simulink model "final_test1"  (Simulink 7.7)
settings: Solver=ode45  StartTime=0.0  StopTime=10.0  RelTol=1e-3
undefined symbols (not defined in the file): des_attributefunction_support, des_figposition
libraries: simeventsattributes2 x107, simeventsserver1 x73, simeventstranslate1 x43, simeventsrouting1 x28, commrandsrc2 x18, simeventsgenerators1 x12, simeventssink1 x9, simeventsqueue1 x6, simulink_extras x1, simeventssignalmanage1 x1
(part 1 of 5)
settings Model: Creator=german  LastModifiedBy=german
settings SimEventsCC: propDiagAttribOutput=1  propDiagFcnCallOutput=1  propDiagStatOutput=0  propDiagChangeAttrib=0

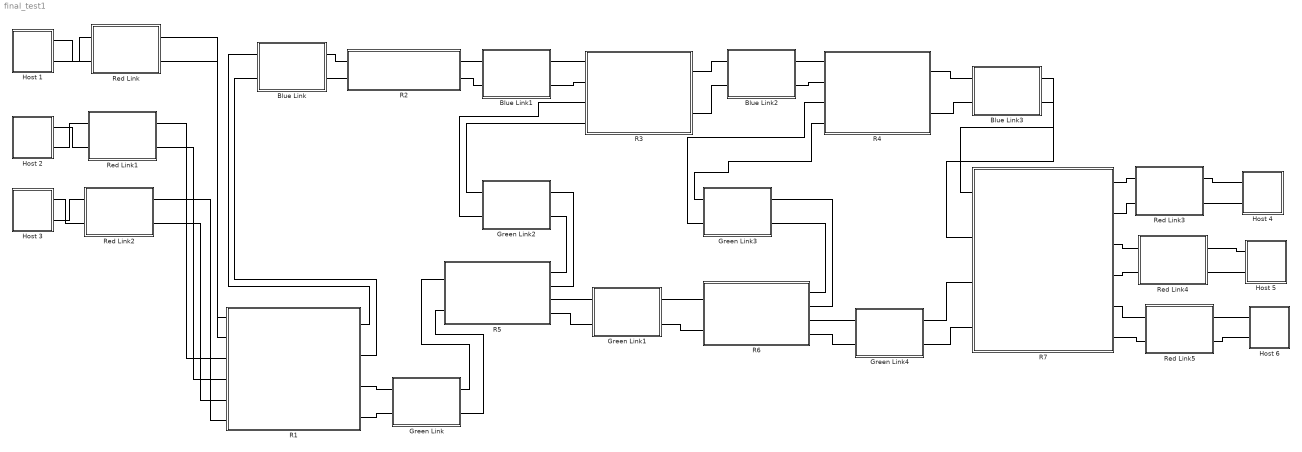
== system final_test1 ==
  Blue Link : Subsystem
  Blue Link1 : Subsystem
  Blue Link2 : Subsystem
  Blue Link3 : Subsystem
  Green Link : Subsystem
  Green Link1 : Subsystem
  Green Link2 : Subsystem
  Green Link3 : Subsystem
  Green Link4 : Subsystem
  Host 1 : Subsystem
  Host 2 : Subsystem
  Host 3 : Subsystem
  Host 4 : Subsystem
  Host 5 : Subsystem
  Host 6 : Subsystem
  R1 : Subsystem
  R2 : Subsystem
  R3 : Subsystem
  R4 : Subsystem
  R5 : Subsystem
  R6 : Subsystem
  R7 : Subsystem
  Red Link : Subsystem
  Red Link1 : Subsystem
  Red Link2 : Subsystem
  Red Link3 : Subsystem
  Red Link4 : Subsystem
  Red Link5 : Subsystem
  connections:
  Red Link/LConn2 -- Host 1/RConn1
  Host 1/RConn2 -- Red Link/LConn1
  Red Link/RConn1 -- R1/LConn1
  R1/LConn2 -- Red Link/RConn2
  Host 2/RConn2 -- Red Link1/LConn1
  Host 2/RConn1 -- Red Link1/LConn2
  Red Link1/RConn1 -- R1/LConn3
  R1/LConn4 -- Red Link1/RConn2
  Host 3/RConn2 -- Red Link2/LConn1
  Red Link2/LConn2 -- Host 3/RConn1
  Red Link2/RConn1 -- R1/LConn6
  Red Link2/RConn2 -- R1/LConn5
  Red Link3/RConn1 -- Host 4/LConn1
  Host 4/LConn2 -- Red Link3/RConn2
  Red Link4/RConn1 -- Host 5/LConn1
  Host 5/LConn2 -- Red Link4/RConn2
  Red Link5/RConn1 -- Host 6/LConn1
  Host 6/LConn2 -- Red Link5/RConn2
  Red Link5/LConn2 -- R7/RConn6
  Red Link5/LConn1 -- R7/RConn5
  Red Link4/LConn2 -- R7/RConn4
  Red Link4/LConn1 -- R7/RConn3
  Red Link3/LConn2 -- R7/RConn2
  Red Link3/LConn1 -- R7/RConn1
  R1/RConn1 -- Blue Link/LConn1
  Blue Link/LConn2 -- R1/RConn2
  Blue Link/RConn1 -- R2/LConn1
  R2/LConn2 -- Blue Link/RConn2
  Blue Link1/RConn1 -- R3/LConn1
  R2/RConn1 -- Blue Link1/LConn1
  R2/RConn2 -- Blue Link1/LConn2
  Blue Link1/RConn2 -- R3/LConn2
  Blue Link2/LConn2 -- R3/RConn2
  Blue Link2/LConn1 -- R3/RConn1
  Blue Link2/RConn1 -- R4/LConn1
  Blue Link2/RConn2 -- R4/LConn2
  R4/RConn1 -- Blue Link3/LConn1
  Blue Link3/LConn2 -- R4/RConn2
  R7/LConn1 -- Blue Link3/RConn1
  Blue Link3/RConn2 -- R7/LConn2
  Green Link/RConn1 -- R5/LConn1
  R1/RConn3 -- Green Link/LConn1
  Green Link/RConn2 -- R5/LConn2
  Green Link/LConn2 -- R1/RConn4
  R5/RConn1 -- Green Link2/RConn2
  R5/RConn2 -- Green Link2/RConn1
  Green Link2/LConn1 -- R3/LConn4
  R3/LConn3 -- Green Link2/LConn2
  R5/RConn3 -- Green Link1/LConn1
  R5/RConn4 -- Green Link1/LConn2
  Green Link1/RConn1 -- R6/LConn1
  Green Link1/RConn2 -- R6/LConn2
  R6/RConn1 -- Green Link3/RConn2
  R6/RConn2 -- Green Link3/RConn1
  Green Link3/LConn1 -- R4/LConn4
  Green Link3/LConn2 -- R4/LConn3
  R6/RConn3 -- Green Link4/LConn1
  R6/RConn4 -- Green Link4/LConn2
  Green Link4/RConn1 -- R7/LConn3
  R7/LConn4 -- Green Link4/RConn2

== system final_test1/Blue Link ==
  Attribute Function : Subsystem  LoadFcn=des_attributefunction_support(gcb,'LoadFcn');  StartFcn=des_attributefunction_support(gcb,'StartFcn');  mask(Attribute Function){OutputNamePrefix=out_}
      mask prompts: OutputNamePrefix "Prefix name"
      settings: CopyFcn=des_attributefunction_support(gcb,'CopyFcn');  OpenFcn=des_attributefunction_support(gcb,'OpenFcn');  ErrorFcn=des_error_redirect
      mask Help: helpview(simeventsbhelp('attributefunction'))
      mask Display: image(des_iconLoad('attribFunction.jpg'),'center');
  Attribute Function1 : Subsystem  LoadFcn=des_attributefunction_support(gcb,'LoadFcn');  StartFcn=des_attributefunction_support(gcb,'StartFcn');  mask(Attribute Function){OutputNamePrefix=out_}
      mask prompts: OutputNamePrefix "Prefix name"
      settings: CopyFcn=des_attributefunction_support(gcb,'CopyFcn');  OpenFcn=des_attributefunction_support(gcb,'OpenFcn');  ErrorFcn=des_error_redirect
      mask Help: helpview(simeventsbhelp('attributefunction'))
      mask Display: image(des_iconLoad('attribFunction.jpg'),'center');
  Infinite Server : simeventsserver1/Infinite Server  SystemSampleTime=-1  ServiceTimeFrom=Dialog  ServiceTime=0.007  AttributeName=ServiceTime  PriorityServiceCompletion=500  EnableTOPort=off  StatNumberDeparted=Off  StatNumberInBlock=Off  StatPendingEntity=Off  StatNumberPending=Off  StatAverageWait=Off  StatNumberTimedout=Off
  Infinite Server1 : simeventsserver1/Infinite Server  SystemSampleTime=-1  ServiceTimeFrom=Dialog  ServiceTime=0.007  AttributeName=ServiceTime  PriorityServiceCompletion=500  EnableTOPort=off  StatNumberDeparted=Off  StatNumberInBlock=Off  StatPendingEntity=Off  StatNumberPending=Off  StatAverageWait=Off  StatNumberTimedout=Off
  Single Server : simeventsserver1/Single Server  SystemSampleTime=-1  ServiceTimeFrom=Attribute  ServiceTime=1  AttributeName=ServiceTime  PriorityServiceCompletion=500  PermitPreemption=off  SortingAttributeName=PriorityAttributeName  SortingDirection=Ascending  WriteToAttribute=off  ResidualAttributeName=ResidualServiceTime  CreateAttribute=on  EnableTOPort=off  StatNumberDeparted=Off  StatNumberInBlock=Off  StatNumberPreempted=Off  StatPendingEntity=Off  StatAverageWait=Off  StatUtilization=Off  StatNumberTimedout=Off
  Single Server1 : simeventsserver1/Single Server  SystemSampleTime=-1  ServiceTimeFrom=Attribute  ServiceTime=1  AttributeName=ServiceTime  PriorityServiceCompletion=500  PermitPreemption=off  SortingAttributeName=PriorityAttributeName  SortingDirection=Ascending  WriteToAttribute=off  ResidualAttributeName=ResidualServiceTime  CreateAttribute=on  EnableTOPort=off  StatNumberDeparted=Off  StatNumberInBlock=Off  StatNumberPreempted=Off  StatPendingEntity=Off  StatAverageWait=Off  StatUtilization=Off  StatNumberTimedout=Off
  Input1 : PMIOPort  Port=1  Side=Left
  Output1 : PMIOPort  Port=2  Side=Right
  Input2 : PMIOPort  Port=3  Side=Right
  Output2 : PMIOPort  Port=4  Side=Left
  connections:
  Attribute Function1/RConn1 -- Single Server1/LConn1
  Input2/RConn1 -- Attribute Function1/LConn1
  Single Server1/RConn1 -- Infinite Server/LConn1
  Single Server/RConn1 -- Infinite Server1/LConn1
  Attribute Function/RConn1 -- Single Server/LConn1
  Output2/RConn1 -- Infinite Server/RConn1
  Output1/RConn1 -- Infinite Server1/RConn1
  Input1/RConn1 -- Attribute Function/LConn1

== system final_test1/Blue Link1 ==
  Attribute Function : Subsystem  LoadFcn=des_attributefunction_support(gcb,'LoadFcn');  StartFcn=des_attributefunction_support(gcb,'StartFcn');  mask(Attribute Function){OutputNamePrefix=out_}
      mask prompts: OutputNamePrefix "Prefix name"
      settings: CopyFcn=des_attributefunction_support(gcb,'CopyFcn');  OpenFcn=des_attributefunction_support(gcb,'OpenFcn');  ErrorFcn=des_error_redirect
      mask Help: helpview(simeventsbhelp('attributefunction'))
      mask Display: image(des_iconLoad('attribFunction.jpg'),'center');
  Attribute Function1 : Subsystem  LoadFcn=des_attributefunction_support(gcb,'LoadFcn');  StartFcn=des_attributefunction_support(gcb,'StartFcn');  mask(Attribute Function){OutputNamePrefix=out_}
      mask prompts: OutputNamePrefix "Prefix name"
      settings: CopyFcn=des_attributefunction_support(gcb,'CopyFcn');  OpenFcn=des_attributefunction_support(gcb,'OpenFcn');  ErrorFcn=des_error_redirect
      mask Help: helpview(simeventsbhelp('attributefunction'))
      mask Display: image(des_iconLoad('attribFunction.jpg'),'center');
  Infinite Server : simeventsserver1/Infinite Server  SystemSampleTime=-1  ServiceTimeFrom=Dialog  ServiceTime=0.007  AttributeName=ServiceTime  PriorityServiceCompletion=500  EnableTOPort=off  StatNumberDeparted=Off  StatNumberInBlock=Off  StatPendingEntity=Off  StatNumberPending=Off  StatAverageWait=Off  StatNumberTimedout=Off
  Infinite Server1 : simeventsserver1/Infinite Server  SystemSampleTime=-1  ServiceTimeFrom=Dialog  ServiceTime=0.007  AttributeName=ServiceTime  PriorityServiceCompletion=500  EnableTOPort=off  StatNumberDeparted=Off  StatNumberInBlock=Off  StatPendingEntity=Off  StatNumberPending=Off  StatAverageWait=Off  StatNumberTimedout=Off
  Single Server : simeventsserver1/Single Server  SystemSampleTime=-1  ServiceTimeFrom=Attribute  ServiceTime=1  AttributeName=ServiceTime  PriorityServiceCompletion=500  PermitPreemption=off  SortingAttributeName=PriorityAttributeName  SortingDirection=Ascending  WriteToAttribute=off  ResidualAttributeName=ResidualServiceTime  CreateAttribute=on  EnableTOPort=off  StatNumberDeparted=Off  StatNumberInBlock=Off  StatNumberPreempted=Off  StatPendingEntity=Off  StatAverageWait=Off  StatUtilization=Off  StatNumberTimedout=Off
  Single Server1 : simeventsserver1/Single Server  SystemSampleTime=-1  ServiceTimeFrom=Attribute  ServiceTime=1  AttributeName=ServiceTime  PriorityServiceCompletion=500  PermitPreemption=off  SortingAttributeName=PriorityAttributeName  SortingDirection=Ascending  WriteToAttribute=off  ResidualAttributeName=ResidualServiceTime  CreateAttribute=on  EnableTOPort=off  StatNumberDeparted=Off  StatNumberInBlock=Off  StatNumberPreempted=Off  StatPendingEntity=Off  StatAverageWait=Off  StatUtilization=Off  StatNumberTimedout=Off
  Input1 : PMIOPort  Port=1  Side=Left
  Output1 : PMIOPort  Port=2  Side=Right
  Input2 : PMIOPort  Port=3  Side=Right
  Output2 : PMIOPort  Port=4  Side=Left
  connections:
  Input1/RConn1 -- Attribute Function/LConn1
  Output1/RConn1 -- Infinite Server1/RConn1
  Output2/RConn1 -- Infinite Server/RConn1
  Attribute Function/RConn1 -- Single Server/LConn1
  Single Server/RConn1 -- Infinite Server1/LConn1
  Single Server1/RConn1 -- Infinite Server/LConn1
  Input2/RConn1 -- Attribute Function1/LConn1
  Attribute Function1/RConn1 -- Single Server1/LConn1

== system final_test1/Blue Link2 ==
  Attribute Function : Subsystem  LoadFcn=des_attributefunction_support(gcb,'LoadFcn');  StartFcn=des_attributefunction_support(gcb,'StartFcn');  mask(Attribute Function){OutputNamePrefix=out_}
      mask prompts: OutputNamePrefix "Prefix name"
      settings: CopyFcn=des_attributefunction_support(gcb,'CopyFcn');  OpenFcn=des_attributefunction_support(gcb,'OpenFcn');  ErrorFcn=des_error_redirect
      mask Help: helpview(simeventsbhelp('attributefunction'))
      mask Display: image(des_iconLoad('attribFunction.jpg'),'center');
  Attribute Function1 : Subsystem  LoadFcn=des_attributefunction_support(gcb,'LoadFcn');  StartFcn=des_attributefunction_support(gcb,'StartFcn');  mask(Attribute Function){OutputNamePrefix=out_}
      mask prompts: OutputNamePrefix "Prefix name"
      settings: CopyFcn=des_attributefunction_support(gcb,'CopyFcn');  OpenFcn=des_attributefunction_support(gcb,'OpenFcn');  ErrorFcn=des_error_redirect
      mask Help: helpview(simeventsbhelp('attributefunction'))
      mask Display: image(des_iconLoad('attribFunction.jpg'),'center');
  Infinite Server : simeventsserver1/Infinite Server  SystemSampleTime=-1  ServiceTimeFrom=Dialog  ServiceTime=0.007  AttributeName=ServiceTime  PriorityServiceCompletion=500  EnableTOPort=off  StatNumberDeparted=Off  StatNumberInBlock=Off  StatPendingEntity=Off  StatNumberPending=Off  StatAverageWait=Off  StatNumberTimedout=Off
  Infinite Server1 : simeventsserver1/Infinite Server  SystemSampleTime=-1  ServiceTimeFrom=Dialog  ServiceTime=0.007  AttributeName=ServiceTime  PriorityServiceCompletion=500  EnableTOPort=off  StatNumberDeparted=Off  StatNumberInBlock=Off  StatPendingEntity=Off  StatNumberPending=Off  StatAverageWait=Off  StatNumberTimedout=Off
  Single Server : simeventsserver1/Single Server  SystemSampleTime=-1  ServiceTimeFrom=Attribute  ServiceTime=1  AttributeName=ServiceTime  PriorityServiceCompletion=500  PermitPreemption=off  SortingAttributeName=PriorityAttributeName  SortingDirection=Ascending  WriteToAttribute=off  ResidualAttributeName=ResidualServiceTime  CreateAttribute=on  EnableTOPort=off  StatNumberDeparted=Off  StatNumberInBlock=Off  StatNumberPreempted=Off  StatPendingEntity=Off  StatAverageWait=Off  StatUtilization=Off  StatNumberTimedout=Off
  Single Server1 : simeventsserver1/Single Server  SystemSampleTime=-1  ServiceTimeFrom=Attribute  ServiceTime=1  AttributeName=ServiceTime  PriorityServiceCompletion=500  PermitPreemption=off  SortingAttributeName=PriorityAttributeName  SortingDirection=Ascending  WriteToAttribute=off  ResidualAttributeName=ResidualServiceTime  CreateAttribute=on  EnableTOPort=off  StatNumberDeparted=Off  StatNumberInBlock=Off  StatNumberPreempted=Off  StatPendingEntity=Off  StatAverageWait=Off  StatUtilization=Off  StatNumberTimedout=Off
  Input1 : PMIOPort  Port=1  Side=Left
  Output1 : PMIOPort  Port=2  Side=Right
  Input2 : PMIOPort  Port=3  Side=Right
  Output2 : PMIOPort  Port=4  Side=Left
  connections:
  Attribute Function1/RConn1 -- Single Server1/LConn1
  Input2/RConn1 -- Attribute Function1/LConn1
  Single Server1/RConn1 -- Infinite Server/LConn1
  Single Server/RConn1 -- Infinite Server1/LConn1
  Attribute Function/RConn1 -- Single Server/LConn1
  Output2/RConn1 -- Infinite Server/RConn1
  Output1/RConn1 -- Infinite Server1/RConn1
  Input1/RConn1 -- Attribute Function/LConn1

== system final_test1/Blue Link3 ==
  Attribute Function : Subsystem  LoadFcn=des_attributefunction_support(gcb,'LoadFcn');  StartFcn=des_attributefunction_support(gcb,'StartFcn');  mask(Attribute Function){OutputNamePrefix=out_}
      mask prompts: OutputNamePrefix "Prefix name"
      settings: CopyFcn=des_attributefunction_support(gcb,'CopyFcn');  OpenFcn=des_attributefunction_support(gcb,'OpenFcn');  ErrorFcn=des_error_redirect
      mask Help: helpview(simeventsbhelp('attributefunction'))
      mask Display: image(des_iconLoad('attribFunction.jpg'),'center');
  Attribute Function1 : Subsystem  LoadFcn=des_attributefunction_support(gcb,'LoadFcn');  StartFcn=des_attributefunction_support(gcb,'StartFcn');  mask(Attribute Function){OutputNamePrefix=out_}
      mask prompts: OutputNamePrefix "Prefix name"
      settings: CopyFcn=des_attributefunction_support(gcb,'CopyFcn');  OpenFcn=des_attributefunction_support(gcb,'OpenFcn');  ErrorFcn=des_error_redirect
      mask Help: helpview(simeventsbhelp('attributefunction'))
      mask Display: image(des_iconLoad('attribFunction.jpg'),'center');
  Infinite Server : simeventsserver1/Infinite Server  SystemSampleTime=-1  ServiceTimeFrom=Dialog  ServiceTime=0.007  AttributeName=ServiceTime  PriorityServiceCompletion=500  EnableTOPort=off  StatNumberDeparted=Off  StatNumberInBlock=Off  StatPendingEntity=Off  StatNumberPending=Off  StatAverageWait=Off  StatNumberTimedout=Off
  Infinite Server1 : simeventsserver1/Infinite Server  SystemSampleTime=-1  ServiceTimeFrom=Dialog  ServiceTime=0.007  AttributeName=ServiceTime  PriorityServiceCompletion=500  EnableTOPort=off  StatNumberDeparted=Off  StatNumberInBlock=Off  StatPendingEntity=Off  StatNumberPending=Off  StatAverageWait=Off  StatNumberTimedout=Off
  Single Server : simeventsserver1/Single Server  SystemSampleTime=-1  ServiceTimeFrom=Attribute  ServiceTime=1  AttributeName=ServiceTime  PriorityServiceCompletion=500  PermitPreemption=off  SortingAttributeName=PriorityAttributeName  SortingDirection=Ascending  WriteToAttribute=off  ResidualAttributeName=ResidualServiceTime  CreateAttribute=on  EnableTOPort=off  StatNumberDeparted=Off  StatNumberInBlock=Off  StatNumberPreempted=Off  StatPendingEntity=Off  StatAverageWait=Off  StatUtilization=Off  StatNumberTimedout=Off
  Single Server1 : simeventsserver1/Single Server  SystemSampleTime=-1  ServiceTimeFrom=Attribute  ServiceTime=1  AttributeName=ServiceTime  PriorityServiceCompletion=500  PermitPreemption=off  SortingAttributeName=PriorityAttributeName  SortingDirection=Ascending  WriteToAttribute=off  ResidualAttributeName=ResidualServiceTime  CreateAttribute=on  EnableTOPort=off  StatNumberDeparted=Off  StatNumberInBlock=Off  StatNumberPreempted=Off  StatPendingEntity=Off  StatAverageWait=Off  StatUtilization=Off  StatNumberTimedout=Off
  Input1 : PMIOPort  Port=1  Side=Left
  Output1 : PMIOPort  Port=2  Side=Right
  Input2 : PMIOPort  Port=3  Side=Right
  Output2 : PMIOPort  Port=4  Side=Left
  connections:
  Input1/RConn1 -- Attribute Function/LConn1
  Output1/RConn1 -- Infinite Server1/RConn1
  Output2/RConn1 -- Infinite Server/RConn1
  Attribute Function/RConn1 -- Single Server/LConn1
  Single Server/RConn1 -- Infinite Server1/LConn1
  Single Server1/RConn1 -- Infinite Server/LConn1
  Input2/RConn1 -- Attribute Function1/LConn1
  Attribute Function1/RConn1 -- Single Server1/LConn1

== system final_test1/Green Link ==
  Attribute Function : Subsystem  LoadFcn=des_attributefunction_support(gcb,'LoadFcn');  StartFcn=des_attributefunction_support(gcb,'StartFcn');  mask(Attribute Function){OutputNamePrefix=out_}
      mask prompts: OutputNamePrefix "Prefix name"
      settings: CopyFcn=des_attributefunction_support(gcb,'CopyFcn');  OpenFcn=des_attributefunction_support(gcb,'OpenFcn');  ErrorFcn=des_error_redirect
      mask Help: helpview(simeventsbhelp('attributefunction'))
      mask Display: image(des_iconLoad('attribFunction.jpg'),'center');
  Attribute Function1 : Subsystem  LoadFcn=des_attributefunction_support(gcb,'LoadFcn');  StartFcn=des_attributefunction_support(gcb,'StartFcn');  mask(Attribute Function){OutputNamePrefix=out_}
      mask prompts: OutputNamePrefix "Prefix name"
      settings: CopyFcn=des_attributefunction_support(gcb,'CopyFcn');  OpenFcn=des_attributefunction_support(gcb,'OpenFcn');  ErrorFcn=des_error_redirect
      mask Help: helpview(simeventsbhelp('attributefunction'))
      mask Display: image(des_iconLoad('attribFunction.jpg'),'center');
  Infinite Server : simeventsserver1/Infinite Server  SystemSampleTime=-1  ServiceTimeFrom=Dialog  ServiceTime=0.003  AttributeName=ServiceTime  PriorityServiceCompletion=500  EnableTOPort=off  StatNumberDeparted=Off  StatNumberInBlock=Off  StatPendingEntity=Off  StatNumberPending=Off  StatAverageWait=Off  StatNumberTimedout=Off
  Infinite Server1 : simeventsserver1/Infinite Server  SystemSampleTime=-1  ServiceTimeFrom=Dialog  ServiceTime=0.003  AttributeName=ServiceTime  PriorityServiceCompletion=500  EnableTOPort=off  StatNumberDeparted=Off  StatNumberInBlock=Off  StatPendingEntity=Off  StatNumberPending=Off  StatAverageWait=Off  StatNumberTimedout=Off
  Single Server : simeventsserver1/Single Server  SystemSampleTime=-1  ServiceTimeFrom=Attribute  ServiceTime=1  AttributeName=ServiceTime  PriorityServiceCompletion=500  PermitPreemption=off  SortingAttributeName=PriorityAttributeName  SortingDirection=Ascending  WriteToAttribute=off  ResidualAttributeName=ResidualServiceTime  CreateAttribute=on  EnableTOPort=off  StatNumberDeparted=Off  StatNumberInBlock=Off  StatNumberPreempted=Off  StatPendingEntity=Off  StatAverageWait=Off  StatUtilization=Off  StatNumberTimedout=Off
  Single Server1 : simeventsserver1/Single Server  SystemSampleTime=-1  ServiceTimeFrom=Attribute  ServiceTime=1  AttributeName=ServiceTime  PriorityServiceCompletion=500  PermitPreemption=off  SortingAttributeName=PriorityAttributeName  SortingDirection=Ascending  WriteToAttribute=off  ResidualAttributeName=ResidualServiceTime  CreateAttribute=on  EnableTOPort=off  StatNumberDeparted=Off  StatNumberInBlock=Off  StatNumberPreempted=Off  StatPendingEntity=Off  StatAverageWait=Off  StatUtilization=Off  StatNumberTimedout=Off
  Input1 : PMIOPort  Port=1  Side=Left
  Output1 : PMIOPort  Port=2  Side=Right
  Input2 : PMIOPort  Port=3  Side=Right
  Output2 : PMIOPort  Port=4  Side=Left
  connections:
  Attribute Function1/RConn1 -- Single Server1/LConn1
  Input2/RConn1 -- Attribute Function1/LConn1
  Single Server1/RConn1 -- Infinite Server/LConn1
  Single Server/RConn1 -- Infinite Server1/LConn1
  Attribute Function/RConn1 -- Single Server/LConn1
  Output2/RConn1 -- Infinite Server/RConn1
  Output1/RConn1 -- Infinite Server1/RConn1
  Input1/RConn1 -- Attribute Function/LConn1

== system final_test1/Green Link1 ==
  Attribute Function : Subsystem  LoadFcn=des_attributefunction_support(gcb,'LoadFcn');  StartFcn=des_attributefunction_support(gcb,'StartFcn');  mask(Attribute Function){OutputNamePrefix=out_}
      mask prompts: OutputNamePrefix "Prefix name"
      settings: CopyFcn=des_attributefunction_support(gcb,'CopyFcn');  OpenFcn=des_attributefunction_support(gcb,'OpenFcn');  ErrorFcn=des_error_redirect
      mask Help: helpview(simeventsbhelp('attributefunction'))
      mask Display: image(des_iconLoad('attribFunction.jpg'),'center');
  Attribute Function1 : Subsystem  LoadFcn=des_attributefunction_support(gcb,'LoadFcn');  StartFcn=des_attributefunction_support(gcb,'StartFcn');  mask(Attribute Function){OutputNamePrefix=out_}
      mask prompts: OutputNamePrefix "Prefix name"
      settings: CopyFcn=des_attributefunction_support(gcb,'CopyFcn');  OpenFcn=des_attributefunction_support(gcb,'OpenFcn');  ErrorFcn=des_error_redirect
      mask Help: helpview(simeventsbhelp('attributefunction'))
      mask Display: image(des_iconLoad('attribFunction.jpg'),'center');
  Infinite Server : simeventsserver1/Infinite Server  SystemSampleTime=-1  ServiceTimeFrom=Dialog  ServiceTime=0.003  AttributeName=ServiceTime  PriorityServiceCompletion=500  EnableTOPort=off  StatNumberDeparted=Off  StatNumberInBlock=Off  StatPendingEntity=Off  StatNumberPending=Off  StatAverageWait=Off  StatNumberTimedout=Off
  Infinite Server1 : simeventsserver1/Infinite Server  SystemSampleTime=-1  ServiceTimeFrom=Dialog  ServiceTime=0.003  AttributeName=ServiceTime  PriorityServiceCompletion=500  EnableTOPort=off  StatNumberDeparted=Off  StatNumberInBlock=Off  StatPendingEntity=Off  StatNumberPending=Off  StatAverageWait=Off  StatNumberTimedout=Off
  Single Server : simeventsserver1/Single Server  SystemSampleTime=-1  ServiceTimeFrom=Attribute  ServiceTime=1  AttributeName=ServiceTime  PriorityServiceCompletion=500  PermitPreemption=off  SortingAttributeName=PriorityAttributeName  SortingDirection=Ascending  WriteToAttribute=off  ResidualAttributeName=ResidualServiceTime  CreateAttribute=on  EnableTOPort=off  StatNumberDeparted=Off  StatNumberInBlock=Off  StatNumberPreempted=Off  StatPendingEntity=Off  StatAverageWait=Off  StatUtilization=Off  StatNumberTimedout=Off
  Single Server1 : simeventsserver1/Single Server  SystemSampleTime=-1  ServiceTimeFrom=Attribute  ServiceTime=1  AttributeName=ServiceTime  PriorityServiceCompletion=500  PermitPreemption=off  SortingAttributeName=PriorityAttributeName  SortingDirection=Ascending  WriteToAttribute=off  ResidualAttributeName=ResidualServiceTime  CreateAttribute=on  EnableTOPort=off  StatNumberDeparted=Off  StatNumberInBlock=Off  StatNumberPreempted=Off  StatPendingEntity=Off  StatAverageWait=Off  StatUtilization=Off  StatNumberTimedout=Off
  Input1 : PMIOPort  Port=1  Side=Left
  Output1 : PMIOPort  Port=2  Side=Right
  Input2 : PMIOPort  Port=3  Side=Right
  Output2 : PMIOPort  Port=4  Side=Left
  connections:
  Input1/RConn1 -- Attribute Function/LConn1
  Output1/RConn1 -- Infinite Server1/RConn1
  Output2/RConn1 -- Infinite Server/RConn1
  Attribute Function/RConn1 -- Single Server/LConn1
  Single Server/RConn1 -- Infinite Server1/LConn1
  Single Server1/RConn1 -- Infinite Server/LConn1
  Input2/RConn1 -- Attribute Function1/LConn1
  Attribute Function1/RConn1 -- Single Server1/LConn1

== system final_test1/Green Link2 ==
  Attribute Function : Subsystem  LoadFcn=des_attributefunction_support(gcb,'LoadFcn');  StartFcn=des_attributefunction_support(gcb,'StartFcn');  mask(Attribute Function){OutputNamePrefix=out_}
      mask prompts: OutputNamePrefix "Prefix name"
      settings: CopyFcn=des_attributefunction_support(gcb,'CopyFcn');  OpenFcn=des_attributefunction_support(gcb,'OpenFcn');  ErrorFcn=des_error_redirect
      mask Help: helpview(simeventsbhelp('attributefunction'))
      mask Display: image(des_iconLoad('attribFunction.jpg'),'center');
  Attribute Function1 : Subsystem  LoadFcn=des_attributefunction_support(gcb,'LoadFcn');  StartFcn=des_attributefunction_support(gcb,'StartFcn');  mask(Attribute Function){OutputNamePrefix=out_}
      mask prompts: OutputNamePrefix "Prefix name"
      settings: CopyFcn=des_attributefunction_support(gcb,'CopyFcn');  OpenFcn=des_attributefunction_support(gcb,'OpenFcn');  ErrorFcn=des_error_redirect
      mask Help: helpview(simeventsbhelp('attributefunction'))
      mask Display: image(des_iconLoad('attribFunction.jpg'),'center');
  Infinite Server : simeventsserver1/Infinite Server  SystemSampleTime=-1  ServiceTimeFrom=Dialog  ServiceTime=0.003  AttributeName=ServiceTime  PriorityServiceCompletion=500  EnableTOPort=off  StatNumberDeparted=Off  StatNumberInBlock=Off  StatPendingEntity=Off  StatNumberPending=Off  StatAverageWait=Off  StatNumberTimedout=Off
  Infinite Server1 : simeventsserver1/Infinite Server  SystemSampleTime=-1  ServiceTimeFrom=Dialog  ServiceTime=0.003  AttributeName=ServiceTime  PriorityServiceCompletion=500  EnableTOPort=off  StatNumberDeparted=Off  StatNumberInBlock=Off  StatPendingEntity=Off  StatNumberPending=Off  StatAverageWait=Off  StatNumberTimedout=Off
  Single Server : simeventsserver1/Single Server  SystemSampleTime=-1  ServiceTimeFrom=Attribute  ServiceTime=1  AttributeName=ServiceTime  PriorityServiceCompletion=500  PermitPreemption=off  SortingAttributeName=PriorityAttributeName  SortingDirection=Ascending  WriteToAttribute=off  ResidualAttributeName=ResidualServiceTime  CreateAttribute=on  EnableTOPort=off  StatNumberDeparted=Off  StatNumberInBlock=Off  StatNumberPreempted=Off  StatPendingEntity=Off  StatAverageWait=Off  StatUtilization=Off  StatNumberTimedout=Off
  Single Server1 : simeventsserver1/Single Server  SystemSampleTime=-1  ServiceTimeFrom=Attribute  ServiceTime=1  AttributeName=ServiceTime  PriorityServiceCompletion=500  PermitPreemption=off  SortingAttributeName=PriorityAttributeName  SortingDirection=Ascending  WriteToAttribute=off  ResidualAttributeName=ResidualServiceTime  CreateAttribute=on  EnableTOPort=off  StatNumberDeparted=Off  StatNumberInBlock=Off  StatNumberPreempted=Off  StatPendingEntity=Off  StatAverageWait=Off  StatUtilization=Off  StatNumberTimedout=Off
  Input1 : PMIOPort  Port=1  Side=Left
  Output1 : PMIOPort  Port=2  Side=Right
  Input2 : PMIOPort  Port=3  Side=Right
  Output2 : PMIOPort  Port=4  Side=Left
  connections:
  Attribute Function1/RConn1 -- Single Server1/LConn1
  Input2/RConn1 -- Attribute Function1/LConn1
  Single Server1/RConn1 -- Infinite Server/LConn1
  Single Server/RConn1 -- Infinite Server1/LConn1
  Attribute Function/RConn1 -- Single Server/LConn1
  Output2/RConn1 -- Infinite Server/RConn1
  Output1/RConn1 -- Infinite Server1/RConn1
  Input1/RConn1 -- Attribute Function/LConn1

== system final_test1/Green Link3 ==
  Attribute Function : Subsystem  LoadFcn=des_attributefunction_support(gcb,'LoadFcn');  StartFcn=des_attributefunction_support(gcb,'StartFcn');  mask(Attribute Function){OutputNamePrefix=out_}
      mask prompts: OutputNamePrefix "Prefix name"
      settings: CopyFcn=des_attributefunction_support(gcb,'CopyFcn');  OpenFcn=des_attributefunction_support(gcb,'OpenFcn');  ErrorFcn=des_error_redirect
      mask Help: helpview(simeventsbhelp('attributefunction'))
      mask Display: image(des_iconLoad('attribFunction.jpg'),'center');
  Attribute Function1 : Subsystem  LoadFcn=des_attributefunction_support(gcb,'LoadFcn');  StartFcn=des_attributefunction_support(gcb,'StartFcn');  mask(Attribute Function){OutputNamePrefix=out_}
      mask prompts: OutputNamePrefix "Prefix name"
      settings: CopyFcn=des_attributefunction_support(gcb,'CopyFcn');  OpenFcn=des_attributefunction_support(gcb,'OpenFcn');  ErrorFcn=des_error_redirect
      mask Help: helpview(simeventsbhelp('attributefunction'))
      mask Display: image(des_iconLoad('attribFunction.jpg'),'center');
  Infinite Server : simeventsserver1/Infinite Server  SystemSampleTime=-1  ServiceTimeFrom=Dialog  ServiceTime=0.003  AttributeName=ServiceTime  PriorityServiceCompletion=500  EnableTOPort=off  StatNumberDeparted=Off  StatNumberInBlock=Off  StatPendingEntity=Off  StatNumberPending=Off  StatAverageWait=Off  StatNumberTimedout=Off
  Infinite Server1 : simeventsserver1/Infinite Server  SystemSampleTime=-1  ServiceTimeFrom=Dialog  ServiceTime=0.003  AttributeName=ServiceTime  PriorityServiceCompletion=500  EnableTOPort=off  StatNumberDeparted=Off  StatNumberInBlock=Off  StatPendingEntity=Off  StatNumberPending=Off  StatAverageWait=Off  StatNumberTimedout=Off
  Single Server : simeventsserver1/Single Server  SystemSampleTime=-1  ServiceTimeFrom=Attribute  ServiceTime=1  AttributeName=ServiceTime  PriorityServiceCompletion=500  PermitPreemption=off  SortingAttributeName=PriorityAttributeName  SortingDirection=Ascending  WriteToAttribute=off  ResidualAttributeName=ResidualServiceTime  CreateAttribute=on  EnableTOPort=off  StatNumberDeparted=Off  StatNumberInBlock=Off  StatNumberPreempted=Off  StatPendingEntity=Off  StatAverageWait=Off  StatUtilization=Off  StatNumberTimedout=Off
  Single Server1 : simeventsserver1/Single Server  SystemSampleTime=-1  ServiceTimeFrom=Attribute  ServiceTime=1  AttributeName=ServiceTime  PriorityServiceCompletion=500  PermitPreemption=off  SortingAttributeName=PriorityAttributeName  SortingDirection=Ascending  WriteToAttribute=off  ResidualAttributeName=ResidualServiceTime  CreateAttribute=on  EnableTOPort=off  StatNumberDeparted=Off  StatNumberInBlock=Off  StatNumberPreempted=Off  StatPendingEntity=Off  StatAverageWait=Off  StatUtilization=Off  StatNumberTimedout=Off
  Input1 : PMIOPort  Port=1  Side=Left
  Output1 : PMIOPort  Port=2  Side=Right
  Input2 : PMIOPort  Port=3  Side=Right
  Output2 : PMIOPort  Port=4  Side=Left
  connections:
  Attribute Function1/RConn1 -- Single Server1/LConn1
  Input2/RConn1 -- Attribute Function1/LConn1
  Single Server1/RConn1 -- Infinite Server/LConn1
  Single Server/RConn1 -- Infinite Server1/LConn1
  Attribute Function/RConn1 -- Single Server/LConn1
  Output2/RConn1 -- Infinite Server/RConn1
  Output1/RConn1 -- Infinite Server1/RConn1
  Input1/RConn1 -- Attribute Function/LConn1

== system final_test1/Green Link4 ==
  Attribute Function : Subsystem  LoadFcn=des_attributefunction_support(gcb,'LoadFcn');  StartFcn=des_attributefunction_support(gcb,'StartFcn');  mask(Attribute Function){OutputNamePrefix=out_}
      mask prompts: OutputNamePrefix "Prefix name"
      settings: CopyFcn=des_attributefunction_support(gcb,'CopyFcn');  OpenFcn=des_attributefunction_support(gcb,'OpenFcn');  ErrorFcn=des_error_redirect
      mask Help: helpview(simeventsbhelp('attributefunction'))
      mask Display: image(des_iconLoad('attribFunction.jpg'),'center');
  Attribute Function1 : Subsystem  LoadFcn=des_attributefunction_support(gcb,'LoadFcn');  StartFcn=des_attributefunction_support(gcb,'StartFcn');  mask(Attribute Function){OutputNamePrefix=out_}
      mask prompts: OutputNamePrefix "Prefix name"
      settings: CopyFcn=des_attributefunction_support(gcb,'CopyFcn');  OpenFcn=des_attributefunction_support(gcb,'OpenFcn');  ErrorFcn=des_error_redirect
      mask Help: helpview(simeventsbhelp('attributefunction'))
      mask Display: image(des_iconLoad('attribFunction.jpg'),'center');
  Infinite Server : simeventsserver1/Infinite Server  SystemSampleTime=-1  ServiceTimeFrom=Dialog  ServiceTime=0.003  AttributeName=ServiceTime  PriorityServiceCompletion=500  EnableTOPort=off  StatNumberDeparted=Off  StatNumberInBlock=Off  StatPendingEntity=Off  StatNumberPending=Off  StatAverageWait=Off  StatNumberTimedout=Off
  Infinite Server1 : simeventsserver1/Infinite Server  SystemSampleTime=-1  ServiceTimeFrom=Dialog  ServiceTime=0.003  AttributeName=ServiceTime  PriorityServiceCompletion=500  EnableTOPort=off  StatNumberDeparted=Off  StatNumberInBlock=Off  StatPendingEntity=Off  StatNumberPending=Off  StatAverageWait=Off  StatNumberTimedout=Off
  Single Server : simeventsserver1/Single Server  SystemSampleTime=-1  ServiceTimeFrom=Attribute  ServiceTime=1  AttributeName=ServiceTime  PriorityServiceCompletion=500  PermitPreemption=off  SortingAttributeName=PriorityAttributeName  SortingDirection=Ascending  WriteToAttribute=off  ResidualAttributeName=ResidualServiceTime  CreateAttribute=on  EnableTOPort=off  StatNumberDeparted=Off  StatNumberInBlock=Off  StatNumberPreempted=Off  StatPendingEntity=Off  StatAverageWait=Off  StatUtilization=Off  StatNumberTimedout=Off
  Single Server1 : simeventsserver1/Single Server  SystemSampleTime=-1  ServiceTimeFrom=Attribute  ServiceTime=1  AttributeName=ServiceTime  PriorityServiceCompletion=500  PermitPreemption=off  SortingAttributeName=PriorityAttributeName  SortingDirection=Ascending  WriteToAttribute=off  ResidualAttributeName=ResidualServiceTime  CreateAttribute=on  EnableTOPort=off  StatNumberDeparted=Off  StatNumberInBlock=Off  StatNumberPreempted=Off  StatPendingEntity=Off  StatAverageWait=Off  StatUtilization=Off  StatNumberTimedout=Off
  Input1 : PMIOPort  Port=1  Side=Left
  Output1 : PMIOPort  Port=2  Side=Right
  Input2 : PMIOPort  Port=3  Side=Right
  Output2 : PMIOPort  Port=4  Side=Left
  connections:
  Input1/RConn1 -- Attribute Function/LConn1
  Output1/RConn1 -- Infinite Server1/RConn1
  Output2/RConn1 -- Infinite Server/RConn1
  Attribute Function/RConn1 -- Single Server/LConn1
  Single Server/RConn1 -- Infinite Server1/LConn1
  Single Server1/RConn1 -- Infinite Server/LConn1
  Input2/RConn1 -- Attribute Function1/LConn1
  Attribute Function1/RConn1 -- Single Server1/LConn1

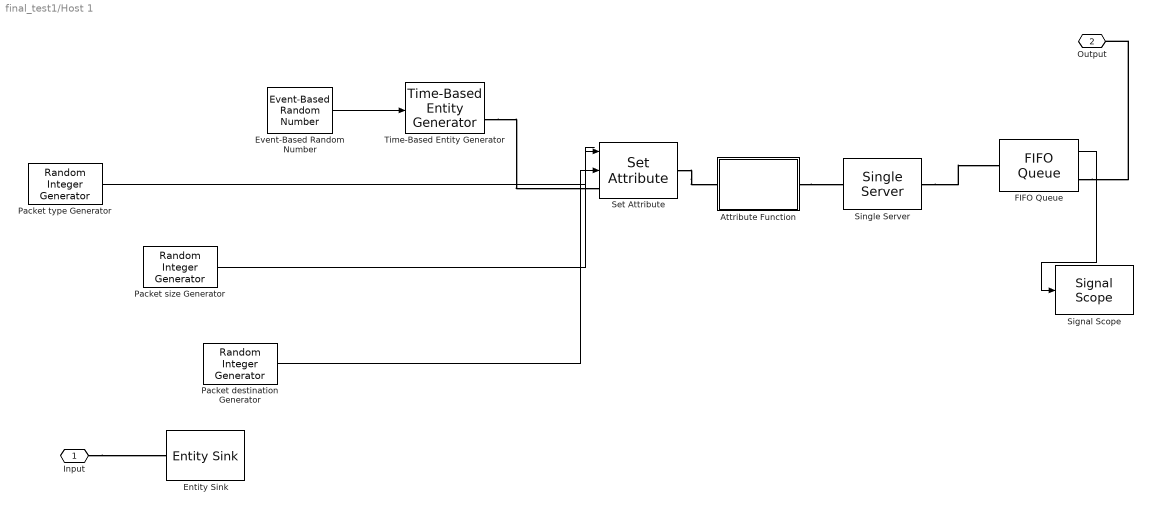
== system final_test1/Host 1 ==
  Attribute Function : Subsystem  LoadFcn=des_attributefunction_support(gcb,'LoadFcn');  StartFcn=des_attributefunction_support(gcb,'StartFcn');  mask(Attribute Function){OutputNamePrefix=out_}
      mask prompts: OutputNamePrefix "Prefix name"
      settings: CopyFcn=des_attributefunction_support(gcb,'CopyFcn');  OpenFcn=des_attributefunction_support(gcb,'OpenFcn');  ErrorFcn=des_error_redirect
      mask Help: helpview(simeventsbhelp('attributefunction'))
      mask Display: image(des_iconLoad('attribFunction.jpg'),'center');
  Entity Sink : simeventssink1/Entity Sink  SystemSampleTime=-1  AvailableForArrivals=on  StatNumberArrived=On
  Event-Based Random Number : simeventsgenerators1/Signal Generators/Event-Based Random Number  SystemSampleTime=-1  distribution=Poisson  meanExp=1  minUnif=1  maxUnif=1  pOneBern=0.25  pSuccessBino=0.5  numTrialBino=1  meanNorm=0  stdNorm=1  minTri=1  maxTri=3  modeTri=2  thresholdLogn=0  scaleLogn=1  shapeLogn=1  pSuccessGeo=0.5  meanPoiss=0.01  thresholdLogl=0  scaleLogl=1  thresholdGam=0  scaleGam=1  shapeGam=1  minBeta=0  maxBeta=1  shape1Beta=1  shape2Beta=1  minUnid=0  maxUnid=1  numValueUnid=2  thresholdWbl=0  scaleWbl=1  shapeWbl=1  valueVecCont=[0 1]  cdfVecCont=[0 1]  valueVecDisc=[0 1]  probVecDisc=[0.5 0.5]  seed=12345  IsProcessed=on  isConnected=1
  FIFO Queue : simeventsqueue1/FIFO Queue  SystemSampleTime=-1  Capacity=25  EnableTOPort=off  StatNumberDeparted=On  StatNumberInBlock=Off  StatPendingEntity=Off  StatAverageWait=Off  StatAverageQueueLength=Off  StatNumberTimedout=Off
  Packet destination Generator : commrandsrc2/Random Integer Generator  SystemSampleTime=-1  mul=6  seed=22  Ts=1  frameBased=off  sampPerFrame=1  orient=off  outDataType=double
  Packet size Generator : commrandsrc2/Random Integer Generator  SystemSampleTime=-1  mul=2  seed=22  Ts=1  frameBased=off  sampPerFrame=1  orient=off  outDataType=double
  Packet type Generator : commrandsrc2/Random Integer Generator  SystemSampleTime=-1  mul=2  seed=37  Ts=1  frameBased=off  sampPerFrame=1  orient=off  outDataType=double
  Set Attribute : simeventsattributes2/Set Attribute  SystemSampleTime=-1  AttributeFrom=Dialog|Signal port|Signal port|Dialog  AttributeName=type|size|dest|from  AttributeTreatAsVector=1|1|1|1  AttributeValue=1|1|4|1  AttributeCreate=on  StatNumberDeparted=Off  EvaluatedAttributeValue={1;[];[];1}
  Signal Scope : simeventssink1/Signal Scope  SystemSampleTime=-1  PlotType=Stair  InputType=Signal  NumInputs=1  AttributeNameY=Count  XInputOptionSignal=Event time  XInputOptionEntity=Event time  AttributeNameX=Count  EnableEntityOutport=on  XMin=0  XMax=10  XLimitExceededOption=Stretch axis limits  YLimitExceededOption=Stretch axis limits  AxisGrid=on  AxisLegend=off  LineDisables=""  LineColors=b  LineStyles=-  LineMarkers=.  OpenScopeAtSimStart=on  Title=""  YLabel=""  XLabel=Time  FigurePosition=des_figposition([5 60 25 25])  AxisZoom=off  DataStoreOption=Limited  DataPointsLimit=10000  StatNumberArrived=Off  ShowCountPlotted=off  ShowToolbar=on
      settings: YMin=0  YMax=10
  Single Server : simeventsserver1/Single Server  SystemSampleTime=-1  ServiceTimeFrom=Dialog  ServiceTime=0  AttributeName=ServiceTime  PriorityServiceCompletion=500  PermitPreemption=off  SortingAttributeName=PriorityAttributeName  SortingDirection=Ascending  WriteToAttribute=off  ResidualAttributeName=ResidualServiceTime  CreateAttribute=on  EnableTOPort=off  StatNumberDeparted=Off  StatNumberInBlock=Off  StatNumberPreempted=Off  StatPendingEntity=Off  StatAverageWait=Off  StatUtilization=Off  StatNumberTimedout=Off
  Time-Based Entity Generator : simeventsgenerators1/Entity Generators/Time-Based Entity Generator  SystemSampleTime=-1  GenerateEntitiesUpon=Intergeneration time from port t  Distribution=Constant  Minimum=0  Maximum=1  Mean=1  InitialSeed=12345  Period=1  PriorityEntityGeneration=300  GenerateEntityAtSimulationStart=on  ResponseWhenBlocked=Pause generation  ResponseWhenUnblocked=Immediate restart  EntityType=Standard  StatNumberDeparted=On  StatPendingEntity=Off  StatAverageIntergenerationTime=Off
  Input : PMIOPort  Port=1  Side=Right
  Output : PMIOPort  Port=2  Side=Right
  wires:
  Event-Based Random Number/1 -> Time-Based Entity Generator/1
  Packet size Generator/1 -> Set Attribute/1
  Packet type Generator/1 -> ?
  Packet destination Generator/1 -> Set Attribute/2
  FIFO Queue/1 -> Signal Scope/1
  connections:
  Time-Based Entity Generator/RConn1 -- Set Attribute/LConn1
  Input/RConn1 -- Entity Sink/LConn1
  Set Attribute/RConn1 -- Attribute Function/LConn1
  FIFO Queue/RConn1 -- Output/RConn1
  Attribute Function/RConn1 -- Single Server/LConn1
  Single Server/RConn1 -- FIFO Queue/LConn1

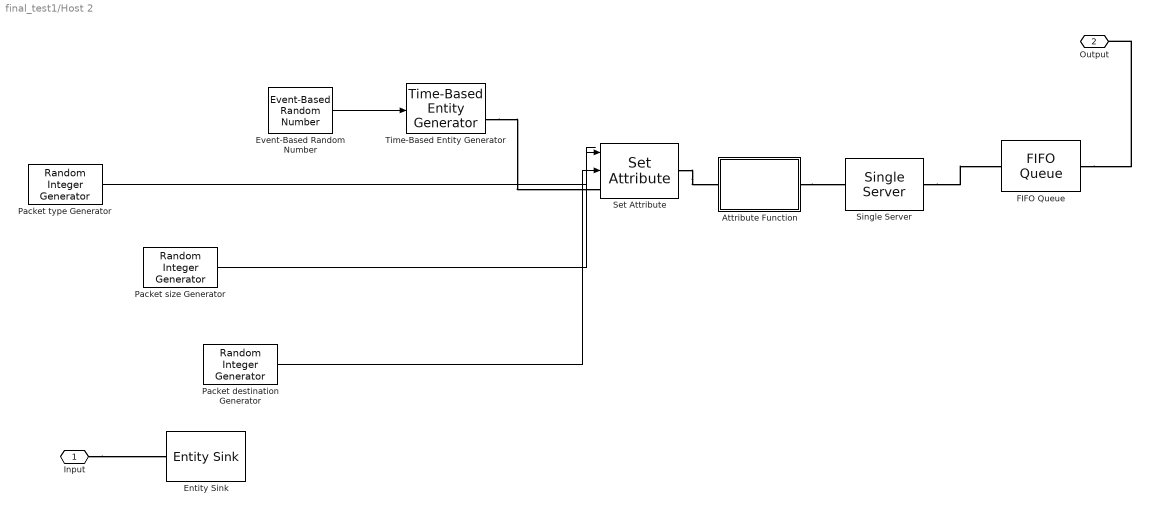
== system final_test1/Host 2 ==
  Attribute Function : Subsystem  LoadFcn=des_attributefunction_support(gcb,'LoadFcn');  StartFcn=des_attributefunction_support(gcb,'StartFcn');  mask(Attribute Function){OutputNamePrefix=out_}
      mask prompts: OutputNamePrefix "Prefix name"
      settings: CopyFcn=des_attributefunction_support(gcb,'CopyFcn');  OpenFcn=des_attributefunction_support(gcb,'OpenFcn');  ErrorFcn=des_error_redirect
      mask Help: helpview(simeventsbhelp('attributefunction'))
      mask Display: image(des_iconLoad('attribFunction.jpg'),'center');
  Entity Sink : simeventssink1/Entity Sink  SystemSampleTime=-1  AvailableForArrivals=on  StatNumberArrived=On
  Event-Based Random Number : simeventsgenerators1/Signal Generators/Event-Based Random Number  SystemSampleTime=-1  distribution=Poisson  meanExp=1  minUnif=1  maxUnif=1  pOneBern=0.25  pSuccessBino=0.5  numTrialBino=1  meanNorm=0  stdNorm=1  minTri=1  maxTri=3  modeTri=2  thresholdLogn=0  scaleLogn=1  shapeLogn=1  pSuccessGeo=0.5  meanPoiss=0.01  thresholdLogl=0  scaleLogl=1  thresholdGam=0  scaleGam=1  shapeGam=1  minBeta=0  maxBeta=1  shape1Beta=1  shape2Beta=1  minUnid=0  maxUnid=1  numValueUnid=2  thresholdWbl=0  scaleWbl=1  shapeWbl=1  valueVecCont=[0 1]  cdfVecCont=[0 1]  valueVecDisc=[0 1]  probVecDisc=[0.5 0.5]  seed=12345  IsProcessed=on  isConnected=1
  FIFO Queue : simeventsqueue1/FIFO Queue  SystemSampleTime=-1  Capacity=25  EnableTOPort=off  StatNumberDeparted=Off  StatNumberInBlock=Off  StatPendingEntity=Off  StatAverageWait=Off  StatAverageQueueLength=Off  StatNumberTimedout=Off
  Packet destination Generator : commrandsrc2/Random Integer Generator  SystemSampleTime=-1  mul=6  seed=22  Ts=1  frameBased=off  sampPerFrame=1  orient=off  outDataType=double
  Packet size Generator : commrandsrc2/Random Integer Generator  SystemSampleTime=-1  mul=2  seed=22  Ts=1  frameBased=off  sampPerFrame=1  orient=off  outDataType=double
  Packet type Generator : commrandsrc2/Random Integer Generator  SystemSampleTime=-1  mul=2  seed=37  Ts=1  frameBased=off  sampPerFrame=1  orient=off  outDataType=double
  Set Attribute : simeventsattributes2/Set Attribute  SystemSampleTime=-1  AttributeFrom=Dialog|Signal port|Signal port|Dialog  AttributeName=type|size|dest|from  AttributeTreatAsVector=1|1|1|1  AttributeValue=1|1|4|2  AttributeCreate=on  StatNumberDeparted=Off  EvaluatedAttributeValue={1;[];[];2}
  Single Server : simeventsserver1/Single Server  SystemSampleTime=-1  ServiceTimeFrom=Dialog  ServiceTime=0  AttributeName=ServiceTime  PriorityServiceCompletion=500  PermitPreemption=off  SortingAttributeName=PriorityAttributeName  SortingDirection=Ascending  WriteToAttribute=off  ResidualAttributeName=ResidualServiceTime  CreateAttribute=on  EnableTOPort=off  StatNumberDeparted=Off  StatNumberInBlock=Off  StatNumberPreempted=Off  StatPendingEntity=Off  StatAverageWait=Off  StatUtilization=Off  StatNumberTimedout=Off
  Time-Based Entity Generator : simeventsgenerators1/Entity Generators/Time-Based Entity Generator  SystemSampleTime=-1  GenerateEntitiesUpon=Intergeneration time from port t  Distribution=Constant  Minimum=0  Maximum=1  Mean=1  InitialSeed=12345  Period=1  PriorityEntityGeneration=300  GenerateEntityAtSimulationStart=on  ResponseWhenBlocked=Pause generation  ResponseWhenUnblocked=Immediate restart  EntityType=Standard  StatNumberDeparted=On  StatPendingEntity=Off  StatAverageIntergenerationTime=Off
  Input : PMIOPort  Port=1  Side=Right
  Output : PMIOPort  Port=2  Side=Right
  wires:
  Packet destination Generator/1 -> Set Attribute/2
  Packet type Generator/1 -> ?
  Packet size Generator/1 -> Set Attribute/1
  Event-Based Random Number/1 -> Time-Based Entity Generator/1
  connections:
  Single Server/RConn1 -- FIFO Queue/LConn1
  Attribute Function/RConn1 -- Single Server/LConn1
  FIFO Queue/RConn1 -- Output/RConn1
  Set Attribute/RConn1 -- Attribute Function/LConn1
  Input/RConn1 -- Entity Sink/LConn1
  Time-Based Entity Generator/RConn1 -- Set Attribute/LConn1

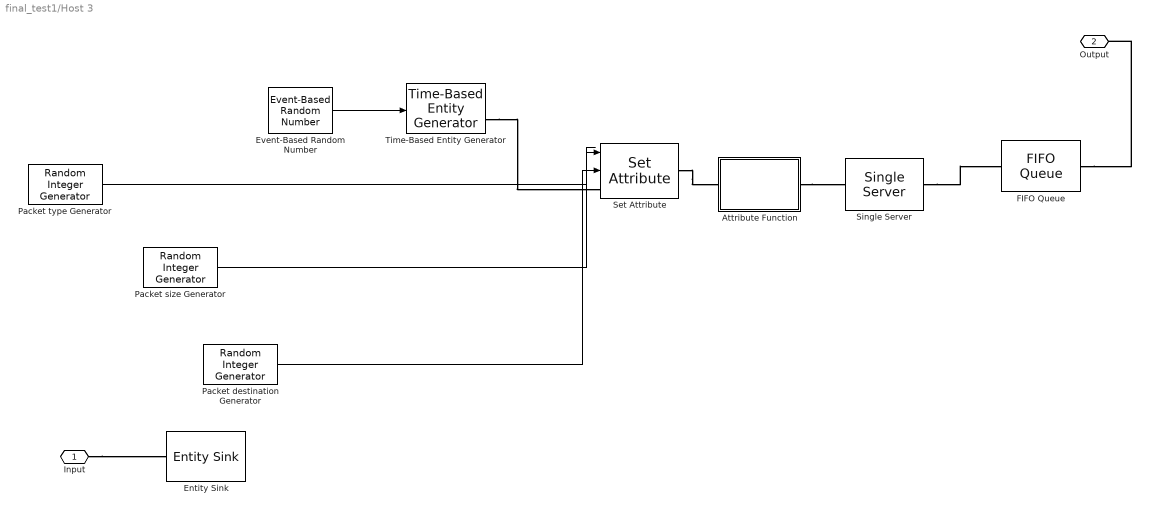
== system final_test1/Host 3 ==
  Attribute Function : Subsystem  LoadFcn=des_attributefunction_support(gcb,'LoadFcn');  StartFcn=des_attributefunction_support(gcb,'StartFcn');  mask(Attribute Function){OutputNamePrefix=out_}
      mask prompts: OutputNamePrefix "Prefix name"
      settings: CopyFcn=des_attributefunction_support(gcb,'CopyFcn');  OpenFcn=des_attributefunction_support(gcb,'OpenFcn');  ErrorFcn=des_error_redirect
      mask Help: helpview(simeventsbhelp('attributefunction'))
      mask Display: image(des_iconLoad('attribFunction.jpg'),'center');
  Entity Sink : simeventssink1/Entity Sink  SystemSampleTime=-1  AvailableForArrivals=on  StatNumberArrived=On
  Event-Based Random Number : simeventsgenerators1/Signal Generators/Event-Based Random Number  SystemSampleTime=-1  distribution=Poisson  meanExp=1  minUnif=1  maxUnif=1  pOneBern=0.25  pSuccessBino=0.5  numTrialBino=1  meanNorm=0  stdNorm=1  minTri=1  maxTri=3  modeTri=2  thresholdLogn=0  scaleLogn=1  shapeLogn=1  pSuccessGeo=0.5  meanPoiss=0.01  thresholdLogl=0  scaleLogl=1  thresholdGam=0  scaleGam=1  shapeGam=1  minBeta=0  maxBeta=1  shape1Beta=1  shape2Beta=1  minUnid=0  maxUnid=1  numValueUnid=2  thresholdWbl=0  scaleWbl=1  shapeWbl=1  valueVecCont=[0 1]  cdfVecCont=[0 1]  valueVecDisc=[0 1]  probVecDisc=[0.5 0.5]  seed=12345  IsProcessed=on  isConnected=1
  FIFO Queue : simeventsqueue1/FIFO Queue  SystemSampleTime=-1  Capacity=25  EnableTOPort=off  StatNumberDeparted=Off  StatNumberInBlock=Off  StatPendingEntity=Off  StatAverageWait=Off  StatAverageQueueLength=Off  StatNumberTimedout=Off
  Packet destination Generator : commrandsrc2/Random Integer Generator  SystemSampleTime=-1  mul=6  seed=22  Ts=1  frameBased=off  sampPerFrame=1  orient=off  outDataType=double
  Packet size Generator : commrandsrc2/Random Integer Generator  SystemSampleTime=-1  mul=2  seed=22  Ts=1  frameBased=off  sampPerFrame=1  orient=off  outDataType=double
  Packet type Generator : commrandsrc2/Random Integer Generator  SystemSampleTime=-1  mul=2  seed=37  Ts=1  frameBased=off  sampPerFrame=1  orient=off  outDataType=double
  Set Attribute : simeventsattributes2/Set Attribute  SystemSampleTime=-1  AttributeFrom=Dialog|Signal port|Signal port|Dialog  AttributeName=type|size|dest|from  AttributeTreatAsVector=1|1|1|1  AttributeValue=1|1|4|3  AttributeCreate=on  StatNumberDeparted=Off  EvaluatedAttributeValue={1;[];[];3}
  Single Server : simeventsserver1/Single Server  SystemSampleTime=-1  ServiceTimeFrom=Dialog  ServiceTime=0  AttributeName=ServiceTime  PriorityServiceCompletion=500  PermitPreemption=off  SortingAttributeName=PriorityAttributeName  SortingDirection=Ascending  WriteToAttribute=off  ResidualAttributeName=ResidualServiceTime  CreateAttribute=on  EnableTOPort=off  StatNumberDeparted=Off  StatNumberInBlock=Off  StatNumberPreempted=Off  StatPendingEntity=Off  StatAverageWait=Off  StatUtilization=Off  StatNumberTimedout=Off
  Time-Based Entity Generator : simeventsgenerators1/Entity Generators/Time-Based Entity Generator  SystemSampleTime=-1  GenerateEntitiesUpon=Intergeneration time from port t  Distribution=Constant  Minimum=0  Maximum=1  Mean=1  InitialSeed=12345  Period=1  PriorityEntityGeneration=300  GenerateEntityAtSimulationStart=on  ResponseWhenBlocked=Pause generation  ResponseWhenUnblocked=Immediate restart  EntityType=Standard  StatNumberDeparted=On  StatPendingEntity=Off  StatAverageIntergenerationTime=Off
  Input : PMIOPort  Port=1  Side=Right
  Output : PMIOPort  Port=2  Side=Right
  wires:
  Event-Based Random Number/1 -> Time-Based Entity Generator/1
  Packet size Generator/1 -> Set Attribute/1
  Packet type Generator/1 -> ?
  Packet destination Generator/1 -> Set Attribute/2
  connections:
  Time-Based Entity Generator/RConn1 -- Set Attribute/LConn1
  Input/RConn1 -- Entity Sink/LConn1
  Set Attribute/RConn1 -- Attribute Function/LConn1
  FIFO Queue/RConn1 -- Output/RConn1
  Attribute Function/RConn1 -- Single Server/LConn1
  Single Server/RConn1 -- FIFO Queue/LConn1
